simulink model "Distribution_vAggregate"  (Simulink 7.9)
settings: Solver=VariableStepDiscrete  StartTime=0.0  StopTime=1000  RelTol=1e-3
libraries: simeventslib x23
(part 1 of 4)
settings Model: Creator=tsprock3  LastModifiedBy=tsprock3
settings DebuggingCC: SimStateOlderReleaseMsg=warning

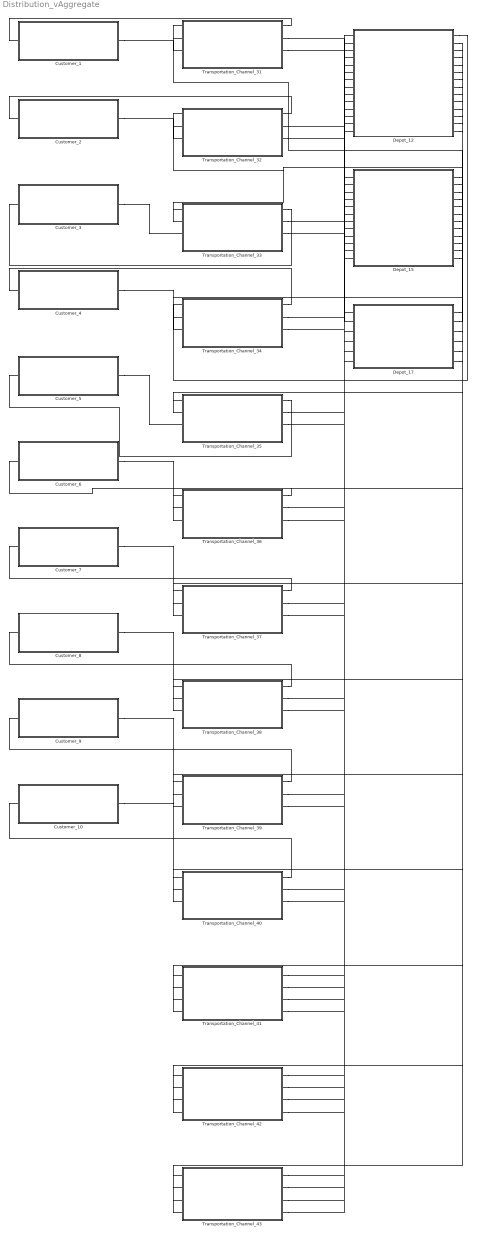
== system Distribution_vAggregate ==
  Customer_1 : Subsystem
  Customer_10 : Subsystem
  Customer_2 : Subsystem
  Customer_3 : Subsystem
  Customer_4 : Subsystem
  Customer_5 : Subsystem
  Customer_6 : Subsystem
  Customer_7 : Subsystem
  Customer_8 : Subsystem
  Customer_9 : Subsystem
  Depot_12 : Subsystem
  Depot_15 : Subsystem
  Depot_17 : Subsystem
  Transportation_Channel_31 : Subsystem
  Transportation_Channel_32 : Subsystem
  Transportation_Channel_33 : Subsystem
  Transportation_Channel_34 : Subsystem
  Transportation_Channel_35 : Subsystem
  Transportation_Channel_36 : Subsystem
  Transportation_Channel_37 : Subsystem
  Transportation_Channel_38 : Subsystem
  Transportation_Channel_39 : Subsystem
  Transportation_Channel_40 : Subsystem
  Transportation_Channel_41 : Subsystem
  Transportation_Channel_42 : Subsystem
  Transportation_Channel_43 : Subsystem
  connections:
  Depot_17/RConn1 -- Transportation_Channel_31/LConn1
  Transportation_Channel_31/RConn1 -- Customer_1/LConn1
  Depot_17/RConn2 -- Transportation_Channel_31/LConn2
  Transportation_Channel_31/RConn2 -- Depot_17/LConn1
  Customer_1/RConn1 -- Transportation_Channel_31/LConn3
  Transportation_Channel_31/RConn3 -- Depot_17/LConn2
  Depot_15/RConn1 -- Transportation_Channel_32/LConn1
  Transportation_Channel_32/RConn1 -- Customer_2/LConn1
  Depot_15/RConn2 -- Transportation_Channel_32/LConn2
  Transportation_Channel_32/RConn2 -- Depot_15/LConn1
  Customer_2/RConn1 -- Transportation_Channel_32/LConn3
  Transportation_Channel_32/RConn3 -- Depot_15/LConn2
  Depot_15/RConn3 -- Transportation_Channel_33/LConn1
  Transportation_Channel_33/RConn1 -- Customer_3/LConn1
  Depot_15/RConn4 -- Transportation_Channel_33/LConn2
  Transportation_Channel_33/RConn2 -- Depot_15/LConn3
  Customer_3/RConn1 -- Transportation_Channel_33/LConn3
  Transportation_Channel_33/RConn3 -- Depot_15/LConn4
  Depot_12/RConn1 -- Transportation_Channel_34/LConn1
  Transportation_Channel_34/RConn1 -- Customer_4/LConn1
  Depot_12/RConn2 -- Transportation_Channel_34/LConn2
  Transportation_Channel_34/RConn2 -- Depot_12/LConn1
  Customer_4/RConn1 -- Transportation_Channel_34/LConn3
  Transportation_Channel_34/RConn3 -- Depot_12/LConn2
  Depot_12/RConn3 -- Transportation_Channel_35/LConn1
  Transportation_Channel_35/RConn1 -- Customer_5/LConn1
  Depot_12/RConn4 -- Transportation_Channel_35/LConn2
  Transportation_Channel_35/RConn2 -- Depot_12/LConn3
  Customer_5/RConn1 -- Transportation_Channel_35/LConn3
  Transportation_Channel_35/RConn3 -- Depot_12/LConn4
  Depot_12/RConn5 -- Transportation_Channel_36/LConn1
  Transportation_Channel_36/RConn1 -- Customer_6/LConn1
  Depot_12/RConn6 -- Transportation_Channel_36/LConn2
  Transportation_Channel_36/RConn2 -- Depot_12/LConn5
  Customer_6/RConn1 -- Transportation_Channel_36/LConn3
  Transportation_Channel_36/RConn3 -- Depot_12/LConn6
  Depot_12/RConn7 -- Transportation_Channel_37/LConn1
  Transportation_Channel_37/RConn1 -- Customer_7/LConn1
  Depot_12/RConn8 -- Transportation_Channel_37/LConn2
  Transportation_Channel_37/RConn2 -- Depot_12/LConn7
  Customer_7/RConn1 -- Transportation_Channel_37/LConn3
  Transportation_Channel_37/RConn3 -- Depot_12/LConn8
  Depot_15/RConn5 -- Transportation_Channel_38/LConn1
  Transportation_Channel_38/RConn1 -- Customer_8/LConn1
  Depot_15/RConn6 -- Transportation_Channel_38/LConn2
  Transportation_Channel_38/RConn2 -- Depot_15/LConn5
  Customer_8/RConn1 -- Transportation_Channel_38/LConn3
  Transportation_Channel_38/RConn3 -- Depot_15/LConn6
  Depot_15/RConn7 -- Transportation_Channel_39/LConn1
  Transportation_Channel_39/RConn1 -- Customer_9/LConn1
  Depot_15/RConn8 -- Transportation_Channel_39/LConn2
  Transportation_Channel_39/RConn2 -- Depot_15/LConn7
  Customer_9/RConn1 -- Transportation_Channel_39/LConn3
  Transportation_Channel_39/RConn3 -- Depot_15/LConn8
  Depot_12/RConn9 -- Transportation_Channel_40/LConn1
  Transportation_Channel_40/RConn1 -- Customer_10/LConn1
  Depot_12/RConn10 -- Transportation_Channel_40/LConn2
  Transportation_Channel_40/RConn2 -- Depot_12/LConn9
  Customer_10/RConn1 -- Transportation_Channel_40/LConn3
  Transportation_Channel_40/RConn3 -- Depot_12/LConn10
  Depot_15/RConn9 -- Transportation_Channel_41/LConn1
  Transportation_Channel_41/RConn1 -- Depot_12/LConn11
  Depot_15/RConn10 -- Transportation_Channel_41/LConn2
  Transportation_Channel_41/RConn2 -- Depot_15/LConn9
  Depot_12/RConn11 -- Transportation_Channel_41/LConn3
  Transportation_Channel_41/RConn3 -- Depot_15/LConn10
  Depot_12/RConn12 -- Transportation_Channel_41/LConn4
  Transportation_Channel_41/RConn4 -- Depot_12/LConn12
  Depot_17/RConn3 -- Transportation_Channel_42/LConn1
  Transportation_Channel_42/RConn1 -- Depot_12/LConn13
  Depot_17/RConn4 -- Transportation_Channel_42/LConn2
  Transportation_Channel_42/RConn2 -- Depot_17/LConn3
  Depot_12/RConn13 -- Transportation_Channel_42/LConn3
  Transportation_Channel_42/RConn3 -- Depot_17/LConn4
  Depot_12/RConn14 -- Transportation_Channel_42/LConn4
  Transportation_Channel_42/RConn4 -- Depot_12/LConn14
  Depot_17/RConn5 -- Transportation_Channel_43/LConn1
  Transportation_Channel_43/RConn1 -- Depot_15/LConn11
  Depot_17/RConn6 -- Transportation_Channel_43/LConn2
  Transportation_Channel_43/RConn2 -- Depot_17/LConn5
  Depot_15/RConn11 -- Transportation_Channel_43/LConn3
  Transportation_Channel_43/RConn3 -- Depot_17/LConn6
  Depot_15/RConn12 -- Transportation_Channel_43/LConn4
  Transportation_Channel_43/RConn4 -- Depot_15/LConn12

== system Distribution_vAggregate/Customer_1 ==
  Commodity_1 : Subsystem  mask{Mean=2000/340, AttributeValue=[1  17  15   2   0   0]|1|2|1}
      mask prompts: Mean "Frequency"; AttributeValue "Attributes"
  Commodity_2 : Subsystem  mask{Mean=2000/473, AttributeValue=[1  17  15   3   0   0]|1|3|1}
      mask prompts: Mean "Frequency"; AttributeValue "Attributes"
  Commodity_3 : Subsystem  mask{Mean=2000/355, AttributeValue=[1  17  12   4   0   0]|1|4|1}
      mask prompts: Mean "Frequency"; AttributeValue "Attributes"
  Commodity_4 : Subsystem  mask{Mean=2000/60, AttributeValue=[1  17  12   5   0   0]|1|5|1}
      mask prompts: Mean "Frequency"; AttributeValue "Attributes"
  Commodity_5 : Subsystem  mask{Mean=2000/226, AttributeValue=[1  17  12   6   0   0]|1|6|1}
      mask prompts: Mean "Frequency"; AttributeValue "Attributes"
  Commodity_6 : Subsystem  mask{Mean=2000/331, AttributeValue=[1  17  12   7   0   0]|1|7|1}
      mask prompts: Mean "Frequency"; AttributeValue "Attributes"
  Commodity_7 : Subsystem  mask{Mean=2000/176, AttributeValue=[1  17  15   8   0   0]|1|8|1}
      mask prompts: Mean "Frequency"; AttributeValue "Attributes"
  Commodity_8 : Subsystem  mask{Mean=2000/209, AttributeValue=[1  17  15   9   0   0]|1|9|1}
      mask prompts: Mean "Frequency"; AttributeValue "Attributes"
  Commodity_9 : Subsystem  mask{Mean=2000/417, AttributeValue=[1  17  12  10   0   0]|1|10|1}
      mask prompts: Mean "Frequency"; AttributeValue "Attributes"
  Entity Sink : EntitySink
  Get Attribute : GetAttribute  AttributeName=Origin|Destination|Start  AttributeMissing=Error|Error|Error  AttributeDefaultValue=1|1|1  AttributeTreatAsVector=1|1|1  AttributeSendTiming=After entity departure|After entity departure|After entity departure  EvaluatedDefaultAttributeValue={[];[];[]}
      settings: OutputPortMap=o1,o2,o3
  Get Attribute1 : GetAttribute  AttributeName=Route  EvaluatedDefaultAttributeValue={[]}
      settings: OutputPortMap=o1
  IN_Commodity : PathCombiner  NumberInputPorts=9
  IN_Shipment : PathCombiner  NumberInputPorts=1
  Lookup : Constant  Value=[17]
  MATLAB Function : MATLAB Function  TreatAsAtomicUnit=on
  Mux : Mux  Inputs=3
  Node_ID : Constant
  OUT_Shipment : OutputSwitch  NumberOutputPorts=1  SwitchingCriterion=From signal port p  AttributeName=Customer
  Shipment_Metrics : simeventslib/SimEvents Sinks/Discrete Event Signal to Workspace  VariableName=Customer_1  SaveFormat=Structure With Time  isMonitorOnly=off  isRecordIC=off
  Single Server : SingleServer  ServiceTime=0
  Timed to Evnt Signal : TimedToEventSignal
  Timed to Evnt Signal1 : TimedToEventSignal
  IN_Shipment_1 : PMIOPort  Port=1  Side=Left
  OUT_Shipment_1 : PMIOPort  Port=2  Side=Right
  wires:
  Timed to Evnt Signal1/1 -> MATLAB Function/3(lookup)
  Lookup/1 -> Timed to Evnt Signal1/1
  Timed to Evnt Signal/1 -> MATLAB Function/2(current)
  Get Attribute1/1 -> MATLAB Function/1(route)
  MATLAB Function/1(next) -> OUT_Shipment/1
  Node_ID/1 -> Timed to Evnt Signal/1
  Mux/1 -> Shipment_Metrics/1
  Get Attribute/3 -> Mux/3
  Get Attribute/2 -> Mux/2
  Get Attribute/1 -> Mux/1
  connections:
  Single Server/RConn1 -- OUT_Shipment/LConn1
  Get Attribute1/RConn1 -- Single Server/LConn1
  IN_Commodity/RConn1 -- Get Attribute1/LConn1
  Get Attribute/LConn1 -- IN_Shipment/RConn1
  Entity Sink/LConn1 -- Get Attribute/RConn1
  IN_Shipment/LConn1 -- IN_Shipment_1/RConn1
  OUT_Shipment/RConn1 -- OUT_Shipment_1/RConn1
  Commodity_1/RConn1 -- IN_Commodity/LConn1
  Commodity_2/RConn1 -- IN_Commodity/LConn2
  Commodity_3/RConn1 -- IN_Commodity/LConn3
  Commodity_4/RConn1 -- IN_Commodity/LConn4
  Commodity_5/RConn1 -- IN_Commodity/LConn5
  Commodity_6/RConn1 -- IN_Commodity/LConn6
  Commodity_7/RConn1 -- IN_Commodity/LConn7
  Commodity_8/RConn1 -- IN_Commodity/LConn8
  Commodity_9/RConn1 -- IN_Commodity/LConn9

== system Distribution_vAggregate/Customer_10 ==
  Commodity_82 : Subsystem  mask{Mean=2000/308, AttributeValue=[10  12  17   1   0   0]|10|1|1}
      mask prompts: Mean "Frequency"; AttributeValue "Attributes"
  Commodity_83 : Subsystem  mask{Mean=2000/25, AttributeValue=[10  12  15   2   0   0]|10|2|1}
      mask prompts: Mean "Frequency"; AttributeValue "Attributes"
  Commodity_84 : Subsystem  mask{Mean=2000/97, AttributeValue=[10  12  15   3   0   0]|10|3|1}
      mask prompts: Mean "Frequency"; AttributeValue "Attributes"
  Commodity_85 : Subsystem  mask{Mean=2000/103, AttributeValue=[10  12   4   0   0   0]|10|4|1}
      mask prompts: Mean "Frequency"; AttributeValue "Attributes"
  Commodity_86 : Subsystem  mask{Mean=2000/95, AttributeValue=[10  12   5   0   0   0]|10|5|1}
      mask prompts: Mean "Frequency"; AttributeValue "Attributes"
  Commodity_87 : Subsystem  mask{Mean=2000/318, AttributeValue=[10  12   6   0   0   0]|10|6|1}
      mask prompts: Mean "Frequency"; AttributeValue "Attributes"
  Commodity_88 : Subsystem  mask{Mean=2000/270, AttributeValue=[10  12   7   0   0   0]|10|7|1}
      mask prompts: Mean "Frequency"; AttributeValue "Attributes"
  Commodity_89 : Subsystem  mask{Mean=2000/250, AttributeValue=[10  12  15   8   0   0]|10|8|1}
      mask prompts: Mean "Frequency"; AttributeValue "Attributes"
  Commodity_90 : Subsystem  mask{Mean=2000/223, AttributeValue=[10  12  15   9   0   0]|10|9|1}
      mask prompts: Mean "Frequency"; AttributeValue "Attributes"
  Entity Sink : EntitySink
  Get Attribute : GetAttribute  AttributeName=Origin|Destination|Start  AttributeMissing=Error|Error|Error  AttributeDefaultValue=1|1|1  AttributeTreatAsVector=1|1|1  AttributeSendTiming=After entity departure|After entity departure|After entity departure  EvaluatedDefaultAttributeValue={[];[];[]}
      settings: OutputPortMap=o1,o2,o3
  Get Attribute1 : GetAttribute  AttributeName=Route  EvaluatedDefaultAttributeValue={[]}
      settings: OutputPortMap=o1
  IN_Commodity : PathCombiner  NumberInputPorts=9
  IN_Shipment : PathCombiner  NumberInputPorts=1
  Lookup : Constant  Value=[12]
  MATLAB Function : MATLAB Function  TreatAsAtomicUnit=on
  Mux : Mux  Inputs=3
  Node_ID : Constant  Value=10
  OUT_Shipment : OutputSwitch  NumberOutputPorts=1  SwitchingCriterion=From signal port p  AttributeName=Customer
  Shipment_Metrics : simeventslib/SimEvents Sinks/Discrete Event Signal to Workspace  VariableName=Customer_10  SaveFormat=Structure With Time  isMonitorOnly=off  isRecordIC=off
  Single Server : SingleServer  ServiceTime=0
  Timed to Evnt Signal : TimedToEventSignal
  Timed to Evnt Signal1 : TimedToEventSignal
  IN_Shipment_1 : PMIOPort  Port=1  Side=Left
  OUT_Shipment_1 : PMIOPort  Port=2  Side=Right
  wires:
  Timed to Evnt Signal1/1 -> MATLAB Function/3(lookup)
  Lookup/1 -> Timed to Evnt Signal1/1
  Timed to Evnt Signal/1 -> MATLAB Function/2(current)
  Get Attribute1/1 -> MATLAB Function/1(route)
  MATLAB Function/1(next) -> OUT_Shipment/1
  Node_ID/1 -> Timed to Evnt Signal/1
  Mux/1 -> Shipment_Metrics/1
  Get Attribute/3 -> Mux/3
  Get Attribute/2 -> Mux/2
  Get Attribute/1 -> Mux/1
  connections:
  Single Server/RConn1 -- OUT_Shipment/LConn1
  Get Attribute1/RConn1 -- Single Server/LConn1
  IN_Commodity/RConn1 -- Get Attribute1/LConn1
  Get Attribute/LConn1 -- IN_Shipment/RConn1
  Entity Sink/LConn1 -- Get Attribute/RConn1
  IN_Shipment/LConn1 -- IN_Shipment_1/RConn1
  OUT_Shipment/RConn1 -- OUT_Shipment_1/RConn1
  Commodity_82/RConn1 -- IN_Commodity/LConn1
  Commodity_83/RConn1 -- IN_Commodity/LConn2
  Commodity_84/RConn1 -- IN_Commodity/LConn3
  Commodity_85/RConn1 -- IN_Commodity/LConn4
  Commodity_86/RConn1 -- IN_Commodity/LConn5
  Commodity_87/RConn1 -- IN_Commodity/LConn6
  Commodity_88/RConn1 -- IN_Commodity/LConn7
  Commodity_89/RConn1 -- IN_Commodity/LConn8
  Commodity_90/RConn1 -- IN_Commodity/LConn9

== system Distribution_vAggregate/Customer_2 ==
  Commodity_10 : Subsystem  mask{Mean=2000/307, AttributeValue=[2  15  17   1   0   0]|2|1|1}
      mask prompts: Mean "Frequency"; AttributeValue "Attributes"
  Commodity_11 : Subsystem  mask{Mean=2000/271, AttributeValue=[2  15   3   0   0   0]|2|3|1}
      mask prompts: Mean "Frequency"; AttributeValue "Attributes"
  Commodity_12 : Subsystem  mask{Mean=2000/133, AttributeValue=[2  15  12   4   0   0]|2|4|1}
      mask prompts: Mean "Frequency"; AttributeValue "Attributes"
  Commodity_13 : Subsystem  mask{Mean=2000/60, AttributeValue=[2  15  12   5   0   0]|2|5|1}
      mask prompts: Mean "Frequency"; AttributeValue "Attributes"
  Commodity_14 : Subsystem  mask{Mean=2000/323, AttributeValue=[2  15  12   6   0   0]|2|6|1}
      mask prompts: Mean "Frequency"; AttributeValue "Attributes"
  Commodity_15 : Subsystem  mask{Mean=2000/320, AttributeValue=[2  15  12   7   0   0]|2|7|1}
      mask prompts: Mean "Frequency"; AttributeValue "Attributes"
  Commodity_16 : Subsystem  mask{Mean=2000/324, AttributeValue=[2  15   8   0   0   0]|2|8|1}
      mask prompts: Mean "Frequency"; AttributeValue "Attributes"
  Commodity_17 : Subsystem  mask{Mean=2000/361, AttributeValue=[2  15   9   0   0   0]|2|9|1}
      mask prompts: Mean "Frequency"; AttributeValue "Attributes"
  Commodity_18 : Subsystem  mask{Mean=2000/497, AttributeValue=[2  15  12  10   0   0]|2|10|1}
      mask prompts: Mean "Frequency"; AttributeValue "Attributes"
  Entity Sink : EntitySink
  Get Attribute : GetAttribute  AttributeName=Origin|Destination|Start  AttributeMissing=Error|Error|Error  AttributeDefaultValue=1|1|1  AttributeTreatAsVector=1|1|1  AttributeSendTiming=After entity departure|After entity departure|After entity departure  EvaluatedDefaultAttributeValue={[];[];[]}
      settings: OutputPortMap=o1,o2,o3
  Get Attribute1 : GetAttribute  AttributeName=Route  EvaluatedDefaultAttributeValue={[]}
      settings: OutputPortMap=o1
  IN_Commodity : PathCombiner  NumberInputPorts=9
  IN_Shipment : PathCombiner  NumberInputPorts=1
  Lookup : Constant  Value=[15]
  MATLAB Function : MATLAB Function  TreatAsAtomicUnit=on
  Mux : Mux  Inputs=3
  Node_ID : Constant  Value=2
  OUT_Shipment : OutputSwitch  NumberOutputPorts=1  SwitchingCriterion=From signal port p  AttributeName=Customer
  Shipment_Metrics : simeventslib/SimEvents Sinks/Discrete Event Signal to Workspace  VariableName=Customer_2  SaveFormat=Structure With Time  isMonitorOnly=off  isRecordIC=off
  Single Server : SingleServer  ServiceTime=0
  Timed to Evnt Signal : TimedToEventSignal
  Timed to Evnt Signal1 : TimedToEventSignal
  IN_Shipment_1 : PMIOPort  Port=1  Side=Left
  OUT_Shipment_1 : PMIOPort  Port=2  Side=Right
  wires:
  Timed to Evnt Signal1/1 -> MATLAB Function/3(lookup)
  Lookup/1 -> Timed to Evnt Signal1/1
  Timed to Evnt Signal/1 -> MATLAB Function/2(current)
  Get Attribute1/1 -> MATLAB Function/1(route)
  MATLAB Function/1(next) -> OUT_Shipment/1
  Node_ID/1 -> Timed to Evnt Signal/1
  Mux/1 -> Shipment_Metrics/1
  Get Attribute/3 -> Mux/3
  Get Attribute/2 -> Mux/2
  Get Attribute/1 -> Mux/1
  connections:
  Single Server/RConn1 -- OUT_Shipment/LConn1
  Get Attribute1/RConn1 -- Single Server/LConn1
  IN_Commodity/RConn1 -- Get Attribute1/LConn1
  Get Attribute/LConn1 -- IN_Shipment/RConn1
  Entity Sink/LConn1 -- Get Attribute/RConn1
  IN_Shipment/LConn1 -- IN_Shipment_1/RConn1
  OUT_Shipment/RConn1 -- OUT_Shipment_1/RConn1
  Commodity_10/RConn1 -- IN_Commodity/LConn1
  Commodity_11/RConn1 -- IN_Commodity/LConn2
  Commodity_12/RConn1 -- IN_Commodity/LConn3
  Commodity_13/RConn1 -- IN_Commodity/LConn4
  Commodity_14/RConn1 -- IN_Commodity/LConn5
  Commodity_15/RConn1 -- IN_Commodity/LConn6
  Commodity_16/RConn1 -- IN_Commodity/LConn7
  Commodity_17/RConn1 -- IN_Commodity/LConn8
  Commodity_18/RConn1 -- IN_Commodity/LConn9

== system Distribution_vAggregate/Customer_3 ==
  Commodity_19 : Subsystem  mask{Mean=2000/53, AttributeValue=[3  15  17   1   0   0]|3|1|1}
      mask prompts: Mean "Frequency"; AttributeValue "Attributes"
  Commodity_20 : Subsystem  mask{Mean=2000/32, AttributeValue=[3  15   2   0   0   0]|3|2|1}
      mask prompts: Mean "Frequency"; AttributeValue "Attributes"
  Commodity_21 : Subsystem  mask{Mean=2000/225, AttributeValue=[3  15  12   4   0   0]|3|4|1}
      mask prompts: Mean "Frequency"; AttributeValue "Attributes"
  Commodity_22 : Subsystem  mask{Mean=2000/382, AttributeValue=[3  15  12   5   0   0]|3|5|1}
      mask prompts: Mean "Frequency"; AttributeValue "Attributes"
  Commodity_23 : Subsystem  mask{Mean=2000/386, AttributeValue=[3  15  12   6   0   0]|3|6|1}
      mask prompts: Mean "Frequency"; AttributeValue "Attributes"
  Commodity_24 : Subsystem  mask{Mean=2000/487, AttributeValue=[3  15  12   7   0   0]|3|7|1}
      mask prompts: Mean "Frequency"; AttributeValue "Attributes"
  Commodity_25 : Subsystem  mask{Mean=2000/70, AttributeValue=[3  15   8   0   0   0]|3|8|1}
      mask prompts: Mean "Frequency"; AttributeValue "Attributes"
  Commodity_26 : Subsystem  mask{Mean=2000/47, AttributeValue=[3  15   9   0   0   0]|3|9|1}
      mask prompts: Mean "Frequency"; AttributeValue "Attributes"
  Commodity_27 : Subsystem  mask{Mean=2000/266, AttributeValue=[3  15  12  10   0   0]|3|10|1}
      mask prompts: Mean "Frequency"; AttributeValue "Attributes"
  Entity Sink : EntitySink
  Get Attribute : GetAttribute  AttributeName=Origin|Destination|Start  AttributeMissing=Error|Error|Error  AttributeDefaultValue=1|1|1  AttributeTreatAsVector=1|1|1  AttributeSendTiming=After entity departure|After entity departure|After entity departure  EvaluatedDefaultAttributeValue={[];[];[]}
      settings: OutputPortMap=o1,o2,o3
  Get Attribute1 : GetAttribute  AttributeName=Route  EvaluatedDefaultAttributeValue={[]}
      settings: OutputPortMap=o1
  IN_Commodity : PathCombiner  NumberInputPorts=9
  IN_Shipment : PathCombiner  NumberInputPorts=1
  Lookup : Constant  Value=[15]
  MATLAB Function : MATLAB Function  TreatAsAtomicUnit=on
  Mux : Mux  Inputs=3
  Node_ID : Constant  Value=3
  OUT_Shipment : OutputSwitch  NumberOutputPorts=1  SwitchingCriterion=From signal port p  AttributeName=Customer
  Shipment_Metrics : simeventslib/SimEvents Sinks/Discrete Event Signal to Workspace  VariableName=Customer_3  SaveFormat=Structure With Time  isMonitorOnly=off  isRecordIC=off
  Single Server : SingleServer  ServiceTime=0
  Timed to Evnt Signal : TimedToEventSignal
  Timed to Evnt Signal1 : TimedToEventSignal
  IN_Shipment_1 : PMIOPort  Port=1  Side=Left
  OUT_Shipment_1 : PMIOPort  Port=2  Side=Right
  wires:
  Timed to Evnt Signal1/1 -> MATLAB Function/3(lookup)
  Lookup/1 -> Timed to Evnt Signal1/1
  Timed to Evnt Signal/1 -> MATLAB Function/2(current)
  Get Attribute1/1 -> MATLAB Function/1(route)
  MATLAB Function/1(next) -> OUT_Shipment/1
  Node_ID/1 -> Timed to Evnt Signal/1
  Mux/1 -> Shipment_Metrics/1
  Get Attribute/3 -> Mux/3
  Get Attribute/2 -> Mux/2
  Get Attribute/1 -> Mux/1
  connections:
  Single Server/RConn1 -- OUT_Shipment/LConn1
  Get Attribute1/RConn1 -- Single Server/LConn1
  IN_Commodity/RConn1 -- Get Attribute1/LConn1
  Get Attribute/LConn1 -- IN_Shipment/RConn1
  Entity Sink/LConn1 -- Get Attribute/RConn1
  IN_Shipment/LConn1 -- IN_Shipment_1/RConn1
  OUT_Shipment/RConn1 -- OUT_Shipment_1/RConn1
  Commodity_19/RConn1 -- IN_Commodity/LConn1
  Commodity_20/RConn1 -- IN_Commodity/LConn2
  Commodity_21/RConn1 -- IN_Commodity/LConn3
  Commodity_22/RConn1 -- IN_Commodity/LConn4
  Commodity_23/RConn1 -- IN_Commodity/LConn5
  Commodity_24/RConn1 -- IN_Commodity/LConn6
  Commodity_25/RConn1 -- IN_Commodity/LConn7
  Commodity_26/RConn1 -- IN_Commodity/LConn8
  Commodity_27/RConn1 -- IN_Commodity/LConn9

== system Distribution_vAggregate/Customer_4 ==
  Commodity_28 : Subsystem  mask{Mean=2000/243, AttributeValue=[4  12  17   1   0   0]|4|1|1}
      mask prompts: Mean "Frequency"; AttributeValue "Attributes"
  Commodity_29 : Subsystem  mask{Mean=2000/336, AttributeValue=[4  12  15   2   0   0]|4|2|1}
      mask prompts: Mean "Frequency"; AttributeValue "Attributes"
  Commodity_30 : Subsystem  mask{Mean=2000/261, AttributeValue=[4  12  15   3   0   0]|4|3|1}
      mask prompts: Mean "Frequency"; AttributeValue "Attributes"
  Commodity_31 : Subsystem  mask{Mean=2000/75, AttributeValue=[4  12   5   0   0   0]|4|5|1}
      mask prompts: Mean "Frequency"; AttributeValue "Attributes"
  Commodity_32 : Subsystem  mask{Mean=2000/132, AttributeValue=[4  12   6   0   0   0]|4|6|1}
      mask prompts: Mean "Frequency"; AttributeValue "Attributes"
  Commodity_33 : Subsystem  mask{Mean=2000/378, AttributeValue=[4  12   7   0   0   0]|4|7|1}
      mask prompts: Mean "Frequency"; AttributeValue "Attributes"
  Commodity_34 : Subsystem  mask{Mean=2000/222, AttributeValue=[4  12  15   8   0   0]|4|8|1}
      mask prompts: Mean "Frequency"; AttributeValue "Attributes"
  Commodity_35 : Subsystem  mask{Mean=2000/180, AttributeValue=[4  12  15   9   0   0]|4|9|1}
      mask prompts: Mean "Frequency"; AttributeValue "Attributes"
  Commodity_36 : Subsystem  mask{Mean=2000/198, AttributeValue=[4  12  10   0   0   0]|4|10|1}
      mask prompts: Mean "Frequency"; AttributeValue "Attributes"
  Entity Sink : EntitySink
  Get Attribute : GetAttribute  AttributeName=Origin|Destination|Start  AttributeMissing=Error|Error|Error  AttributeDefaultValue=1|1|1  AttributeTreatAsVector=1|1|1  AttributeSendTiming=After entity departure|After entity departure|After entity departure  EvaluatedDefaultAttributeValue={[];[];[]}
      settings: OutputPortMap=o1,o2,o3
  Get Attribute1 : GetAttribute  AttributeName=Route  EvaluatedDefaultAttributeValue={[]}
      settings: OutputPortMap=o1
  IN_Commodity : PathCombiner  NumberInputPorts=9
  IN_Shipment : PathCombiner  NumberInputPorts=1
  Lookup : Constant  Value=[12]
  MATLAB Function : MATLAB Function  TreatAsAtomicUnit=on
  Mux : Mux  Inputs=3
  Node_ID : Constant  Value=4
  OUT_Shipment : OutputSwitch  NumberOutputPorts=1  SwitchingCriterion=From signal port p  AttributeName=Customer
  Shipment_Metrics : simeventslib/SimEvents Sinks/Discrete Event Signal to Workspace  VariableName=Customer_4  SaveFormat=Structure With Time  isMonitorOnly=off  isRecordIC=off
  Single Server : SingleServer  ServiceTime=0
  Timed to Evnt Signal : TimedToEventSignal
  Timed to Evnt Signal1 : TimedToEventSignal
  IN_Shipment_1 : PMIOPort  Port=1  Side=Left
  OUT_Shipment_1 : PMIOPort  Port=2  Side=Right
  wires:
  Timed to Evnt Signal1/1 -> MATLAB Function/3(lookup)
  Lookup/1 -> Timed to Evnt Signal1/1
  Timed to Evnt Signal/1 -> MATLAB Function/2(current)
  Get Attribute1/1 -> MATLAB Function/1(route)
  MATLAB Function/1(next) -> OUT_Shipment/1
  Node_ID/1 -> Timed to Evnt Signal/1
  Mux/1 -> Shipment_Metrics/1
  Get Attribute/3 -> Mux/3
  Get Attribute/2 -> Mux/2
  Get Attribute/1 -> Mux/1
  connections:
  Single Server/RConn1 -- OUT_Shipment/LConn1
  Get Attribute1/RConn1 -- Single Server/LConn1
  IN_Commodity/RConn1 -- Get Attribute1/LConn1
  Get Attribute/LConn1 -- IN_Shipment/RConn1
  Entity Sink/LConn1 -- Get Attribute/RConn1
  IN_Shipment/LConn1 -- IN_Shipment_1/RConn1
  OUT_Shipment/RConn1 -- OUT_Shipment_1/RConn1
  Commodity_28/RConn1 -- IN_Commodity/LConn1
  Commodity_29/RConn1 -- IN_Commodity/LConn2
  Commodity_30/RConn1 -- IN_Commodity/LConn3
  Commodity_31/RConn1 -- IN_Commodity/LConn4
  Commodity_32/RConn1 -- IN_Commodity/LConn5
  Commodity_33/RConn1 -- IN_Commodity/LConn6
  Commodity_34/RConn1 -- IN_Commodity/LConn7
  Commodity_35/RConn1 -- IN_Commodity/LConn8
  Commodity_36/RConn1 -- IN_Commodity/LConn9

== system Distribution_vAggregate/Customer_5 ==
  Commodity_37 : Subsystem  mask{Mean=2000/353, AttributeValue=[5  12  17   1   0   0]|5|1|1}
      mask prompts: Mean "Frequency"; AttributeValue "Attributes"
  Commodity_38 : Subsystem  mask{Mean=2000/10, AttributeValue=[5  12  15   2   0   0]|5|2|1}
      mask prompts: Mean "Frequency"; AttributeValue "Attributes"
  Commodity_39 : Subsystem  mask{Mean=2000/213, AttributeValue=[5  12  15   3   0   0]|5|3|1}
      mask prompts: Mean "Frequency"; AttributeValue "Attributes"
  Commodity_40 : Subsystem  mask{Mean=2000/99, AttributeValue=[5  12   4   0   0   0]|5|4|1}
      mask prompts: Mean "Frequency"; AttributeValue "Attributes"
  Commodity_41 : Subsystem  mask{Mean=2000/215, AttributeValue=[5  12   6   0   0   0]|5|6|1}
      mask prompts: Mean "Frequency"; AttributeValue "Attributes"
  Commodity_42 : Subsystem  mask{Mean=2000/196, AttributeValue=[5  12   7   0   0   0]|5|7|1}
      mask prompts: Mean "Frequency"; AttributeValue "Attributes"
  Commodity_43 : Subsystem  mask{Mean=2000/199, AttributeValue=[5  12  15   8   0   0]|5|8|1}
      mask prompts: Mean "Frequency"; AttributeValue "Attributes"
  Commodity_44 : Subsystem  mask{Mean=2000/378, AttributeValue=[5  12  15   9   0   0]|5|9|1}
      mask prompts: Mean "Frequency"; AttributeValue "Attributes"
  Commodity_45 : Subsystem  mask{Mean=2000/109, AttributeValue=[5  12  10   0   0   0]|5|10|1}
      mask prompts: Mean "Frequency"; AttributeValue "Attributes"
  Entity Sink : EntitySink
  Get Attribute : GetAttribute  AttributeName=Origin|Destination|Start  AttributeMissing=Error|Error|Error  AttributeDefaultValue=1|1|1  AttributeTreatAsVector=1|1|1  AttributeSendTiming=After entity departure|After entity departure|After entity departure  EvaluatedDefaultAttributeValue={[];[];[]}
      settings: OutputPortMap=o1,o2,o3
  Get Attribute1 : GetAttribute  AttributeName=Route  EvaluatedDefaultAttributeValue={[]}
      settings: OutputPortMap=o1
  IN_Commodity : PathCombiner  NumberInputPorts=9
  IN_Shipment : PathCombiner  NumberInputPorts=1
  Lookup : Constant  Value=[12]
  MATLAB Function : MATLAB Function  TreatAsAtomicUnit=on
  Mux : Mux  Inputs=3
  Node_ID : Constant  Value=5
  OUT_Shipment : OutputSwitch  NumberOutputPorts=1  SwitchingCriterion=From signal port p  AttributeName=Customer
  Shipment_Metrics : simeventslib/SimEvents Sinks/Discrete Event Signal to Workspace  VariableName=Customer_5  SaveFormat=Structure With Time  isMonitorOnly=off  isRecordIC=off
  Single Server : SingleServer  ServiceTime=0
  Timed to Evnt Signal : TimedToEventSignal
  Timed to Evnt Signal1 : TimedToEventSignal
  IN_Shipment_1 : PMIOPort  Port=1  Side=Left
  OUT_Shipment_1 : PMIOPort  Port=2  Side=Right
  wires:
  Timed to Evnt Signal1/1 -> MATLAB Function/3(lookup)
  Lookup/1 -> Timed to Evnt Signal1/1
  Timed to Evnt Signal/1 -> MATLAB Function/2(current)
  Get Attribute1/1 -> MATLAB Function/1(route)
  MATLAB Function/1(next) -> OUT_Shipment/1
  Node_ID/1 -> Timed to Evnt Signal/1
  Mux/1 -> Shipment_Metrics/1
  Get Attribute/3 -> Mux/3
  Get Attribute/2 -> Mux/2
  Get Attribute/1 -> Mux/1
  connections:
  Single Server/RConn1 -- OUT_Shipment/LConn1
  Get Attribute1/RConn1 -- Single Server/LConn1
  IN_Commodity/RConn1 -- Get Attribute1/LConn1
  Get Attribute/LConn1 -- IN_Shipment/RConn1
  Entity Sink/LConn1 -- Get Attribute/RConn1
  IN_Shipment/LConn1 -- IN_Shipment_1/RConn1
  OUT_Shipment/RConn1 -- OUT_Shipment_1/RConn1
  Commodity_37/RConn1 -- IN_Commodity/LConn1
  Commodity_38/RConn1 -- IN_Commodity/LConn2
  Commodity_39/RConn1 -- IN_Commodity/LConn3
  Commodity_40/RConn1 -- IN_Commodity/LConn4
  Commodity_41/RConn1 -- IN_Commodity/LConn5
  Commodity_42/RConn1 -- IN_Commodity/LConn6
  Commodity_43/RConn1 -- IN_Commodity/LConn7
  Commodity_44/RConn1 -- IN_Commodity/LConn8
  Commodity_45/RConn1 -- IN_Commodity/LConn9

== system Distribution_vAggregate/Customer_6 ==
  Commodity_46 : Subsystem  mask{Mean=2000/475, AttributeValue=[6  12  17   1   0   0]|6|1|1}
      mask prompts: Mean "Frequency"; AttributeValue "Attributes"
  Commodity_47 : Subsystem  mask{Mean=2000/336, AttributeValue=[6  12  15   2   0   0]|6|2|1}
      mask prompts: Mean "Frequency"; AttributeValue "Attributes"
  Commodity_48 : Subsystem  mask{Mean=2000/417, AttributeValue=[6  12  15   3   0   0]|6|3|1}
      mask prompts: Mean "Frequency"; AttributeValue "Attributes"
  Commodity_49 : Subsystem  mask{Mean=2000/84, AttributeValue=[6  12   4   0   0   0]|6|4|1}
      mask prompts: Mean "Frequency"; AttributeValue "Attributes"
  Commodity_50 : Subsystem  mask{Mean=2000/495, AttributeValue=[6  12   5   0   0   0]|6|5|1}
      mask prompts: Mean "Frequency"; AttributeValue "Attributes"
  Commodity_51 : Subsystem  mask{Mean=2000/443, AttributeValue=[6  12   7   0   0   0]|6|7|1}
      mask prompts: Mean "Frequency"; AttributeValue "Attributes"
  Commodity_52 : Subsystem  mask{Mean=2000/78, AttributeValue=[6  12  15   8   0   0]|6|8|1}
      mask prompts: Mean "Frequency"; AttributeValue "Attributes"
  Commodity_53 : Subsystem  mask{Mean=2000/204, AttributeValue=[6  12  15   9   0   0]|6|9|1}
      mask prompts: Mean "Frequency"; AttributeValue "Attributes"
  Commodity_54 : Subsystem  mask{Mean=2000/413, AttributeValue=[6  12  10   0   0   0]|6|10|1}
      mask prompts: Mean "Frequency"; AttributeValue "Attributes"
  Entity Sink : EntitySink
  Get Attribute : GetAttribute  AttributeName=Origin|Destination|Start  AttributeMissing=Error|Error|Error  AttributeDefaultValue=1|1|1  AttributeTreatAsVector=1|1|1  AttributeSendTiming=After entity departure|After entity departure|After entity departure  EvaluatedDefaultAttributeValue={[];[];[]}
      settings: OutputPortMap=o1,o2,o3
  Get Attribute1 : GetAttribute  AttributeName=Route  EvaluatedDefaultAttributeValue={[]}
      settings: OutputPortMap=o1
  IN_Commodity : PathCombiner  NumberInputPorts=9
  IN_Shipment : PathCombiner  NumberInputPorts=1
  Lookup : Constant  Value=[12]
  MATLAB Function : MATLAB Function  TreatAsAtomicUnit=on
  Mux : Mux  Inputs=3
  Node_ID : Constant  Value=6
  OUT_Shipment : OutputSwitch  NumberOutputPorts=1  SwitchingCriterion=From signal port p  AttributeName=Customer
  Shipment_Metrics : simeventslib/SimEvents Sinks/Discrete Event Signal to Workspace  VariableName=Customer_6  SaveFormat=Structure With Time  isMonitorOnly=off  isRecordIC=off
  Single Server : SingleServer  ServiceTime=0
  Timed to Evnt Signal : TimedToEventSignal
  Timed to Evnt Signal1 : TimedToEventSignal
  IN_Shipment_1 : PMIOPort  Port=1  Side=Left
  OUT_Shipment_1 : PMIOPort  Port=2  Side=Right
  wires:
  Timed to Evnt Signal1/1 -> MATLAB Function/3(lookup)
  Lookup/1 -> Timed to Evnt Signal1/1
  Timed to Evnt Signal/1 -> MATLAB Function/2(current)
  Get Attribute1/1 -> MATLAB Function/1(route)
  MATLAB Function/1(next) -> OUT_Shipment/1
  Node_ID/1 -> Timed to Evnt Signal/1
  Mux/1 -> Shipment_Metrics/1
  Get Attribute/3 -> Mux/3
  Get Attribute/2 -> Mux/2
  Get Attribute/1 -> Mux/1
  connections:
  Single Server/RConn1 -- OUT_Shipment/LConn1
  Get Attribute1/RConn1 -- Single Server/LConn1
  IN_Commodity/RConn1 -- Get Attribute1/LConn1
  Get Attribute/LConn1 -- IN_Shipment/RConn1
  Entity Sink/LConn1 -- Get Attribute/RConn1
  IN_Shipment/LConn1 -- IN_Shipment_1/RConn1
  OUT_Shipment/RConn1 -- OUT_Shipment_1/RConn1
  Commodity_46/RConn1 -- IN_Commodity/LConn1
  Commodity_47/RConn1 -- IN_Commodity/LConn2
  Commodity_48/RConn1 -- IN_Commodity/LConn3
  Commodity_49/RConn1 -- IN_Commodity/LConn4
  Commodity_50/RConn1 -- IN_Commodity/LConn5
  Commodity_51/RConn1 -- IN_Commodity/LConn6
  Commodity_52/RConn1 -- IN_Commodity/LConn7
  Commodity_53/RConn1 -- IN_Commodity/LConn8
  Commodity_54/RConn1 -- IN_Commodity/LConn9

== system Distribution_vAggregate/Customer_7 ==
  Commodity_55 : Subsystem  mask{Mean=2000/160, AttributeValue=[7  12  17   1   0   0]|7|1|1}
      mask prompts: Mean "Frequency"; AttributeValue "Attributes"
  Commodity_56 : Subsystem  mask{Mean=2000/45, AttributeValue=[7  12  15   2   0   0]|7|2|1}
      mask prompts: Mean "Frequency"; AttributeValue "Attributes"
  Commodity_57 : Subsystem  mask{Mean=2000/69, AttributeValue=[7  12  15   3   0   0]|7|3|1}
      mask prompts: Mean "Frequency"; AttributeValue "Attributes"
  Commodity_58 : Subsystem  mask{Mean=2000/248, AttributeValue=[7  12   4   0   0   0]|7|4|1}
      mask prompts: Mean "Frequency"; AttributeValue "Attributes"
  Commodity_59 : Subsystem  mask{Mean=2000/248, AttributeValue=[7  12   5   0   0   0]|7|5|1}
      mask prompts: Mean "Frequency"; AttributeValue "Attributes"
  Commodity_60 : Subsystem  mask{Mean=2000/28, AttributeValue=[7  12   6   0   0   0]|7|6|1}
      mask prompts: Mean "Frequency"; AttributeValue "Attributes"
  Commodity_61 : Subsystem  mask{Mean=2000/281, AttributeValue=[7  12  15   8   0   0]|7|8|1}
      mask prompts: Mean "Frequency"; AttributeValue "Attributes"
  Commodity_62 : Subsystem  mask{Mean=2000/349, AttributeValue=[7  12  15   9   0   0]|7|9|1}
      mask prompts: Mean "Frequency"; AttributeValue "Attributes"
  Commodity_63 : Subsystem  mask{Mean=2000/408, AttributeValue=[7  12  10   0   0   0]|7|10|1}
      mask prompts: Mean "Frequency"; AttributeValue "Attributes"
  Entity Sink : EntitySink
  Get Attribute : GetAttribute  AttributeName=Origin|Destination|Start  AttributeMissing=Error|Error|Error  AttributeDefaultValue=1|1|1  AttributeTreatAsVector=1|1|1  AttributeSendTiming=After entity departure|After entity departure|After entity departure  EvaluatedDefaultAttributeValue={[];[];[]}
      settings: OutputPortMap=o1,o2,o3
  Get Attribute1 : GetAttribute  AttributeName=Route  EvaluatedDefaultAttributeValue={[]}
      settings: OutputPortMap=o1
  IN_Commodity : PathCombiner  NumberInputPorts=9
  IN_Shipment : PathCombiner  NumberInputPorts=1
  Lookup : Constant  Value=[12]
  MATLAB Function : MATLAB Function  TreatAsAtomicUnit=on
  Mux : Mux  Inputs=3
  Node_ID : Constant  Value=7
  OUT_Shipment : OutputSwitch  NumberOutputPorts=1  SwitchingCriterion=From signal port p  AttributeName=Customer
  Shipment_Metrics : simeventslib/SimEvents Sinks/Discrete Event Signal to Workspace  VariableName=Customer_7  SaveFormat=Structure With Time  isMonitorOnly=off  isRecordIC=off
  Single Server : SingleServer  ServiceTime=0
  Timed to Evnt Signal : TimedToEventSignal
  Timed to Evnt Signal1 : TimedToEventSignal
  IN_Shipment_1 : PMIOPort  Port=1  Side=Left
  OUT_Shipment_1 : PMIOPort  Port=2  Side=Right
  wires:
  Timed to Evnt Signal1/1 -> MATLAB Function/3(lookup)
  Lookup/1 -> Timed to Evnt Signal1/1
  Timed to Evnt Signal/1 -> MATLAB Function/2(current)
  Get Attribute1/1 -> MATLAB Function/1(route)
  MATLAB Function/1(next) -> OUT_Shipment/1
  Node_ID/1 -> Timed to Evnt Signal/1
  Mux/1 -> Shipment_Metrics/1
  Get Attribute/3 -> Mux/3
  Get Attribute/2 -> Mux/2
  Get Attribute/1 -> Mux/1
  connections:
  Single Server/RConn1 -- OUT_Shipment/LConn1
  Get Attribute1/RConn1 -- Single Server/LConn1
  IN_Commodity/RConn1 -- Get Attribute1/LConn1
  Get Attribute/LConn1 -- IN_Shipment/RConn1
  Entity Sink/LConn1 -- Get Attribute/RConn1
  IN_Shipment/LConn1 -- IN_Shipment_1/RConn1
  OUT_Shipment/RConn1 -- OUT_Shipment_1/RConn1
  Commodity_55/RConn1 -- IN_Commodity/LConn1
  Commodity_56/RConn1 -- IN_Commodity/LConn2
  Commodity_57/RConn1 -- IN_Commodity/LConn3
  Commodity_58/RConn1 -- IN_Commodity/LConn4
  Commodity_59/RConn1 -- IN_Commodity/LConn5
  Commodity_60/RConn1 -- IN_Commodity/LConn6
  Commodity_61/RConn1 -- IN_Commodity/LConn7
  Commodity_62/RConn1 -- IN_Commodity/LConn8
  Commodity_63/RConn1 -- IN_Commodity/LConn9

== system Distribution_vAggregate/Customer_8 ==
  Commodity_64 : Subsystem  mask{Mean=2000/495, AttributeValue=[8  15  17   1   0   0]|8|1|1}
      mask prompts: Mean "Frequency"; AttributeValue "Attributes"
  Commodity_65 : Subsystem  mask{Mean=2000/433, AttributeValue=[8  15   2   0   0   0]|8|2|1}
      mask prompts: Mean "Frequency"; AttributeValue "Attributes"
  Commodity_66 : Subsystem  mask{Mean=2000/495, AttributeValue=[8  15   3   0   0   0]|8|3|1}
      mask prompts: Mean "Frequency"; AttributeValue "Attributes"
  Commodity_67 : Subsystem  mask{Mean=2000/240, AttributeValue=[8  15  12   4   0   0]|8|4|1}
      mask prompts: Mean "Frequency"; AttributeValue "Attributes"
  Commodity_68 : Subsystem  mask{Mean=2000/114, AttributeValue=[8  15  12   5   0   0]|8|5|1}
      mask prompts: Mean "Frequency"; AttributeValue "Attributes"
  Commodity_69 : Subsystem  mask{Mean=2000/451, AttributeValue=[8  15  12   6   0   0]|8|6|1}
      mask prompts: Mean "Frequency"; AttributeValue "Attributes"
  Commodity_70 : Subsystem  mask{Mean=2000/423, AttributeValue=[8  15  12   7   0   0]|8|7|1}
      mask prompts: Mean "Frequency"; AttributeValue "Attributes"
  Commodity_71 : Subsystem  mask{Mean=2000/293, AttributeValue=[8  15   9   0   0   0]|8|9|1}
      mask prompts: Mean "Frequency"; AttributeValue "Attributes"
  Commodity_72 : Subsystem  mask{Mean=2000/334, AttributeValue=[8  15  12  10   0   0]|8|10|1}
      mask prompts: Mean "Frequency"; AttributeValue "Attributes"
  Entity Sink : EntitySink
  Get Attribute : GetAttribute  AttributeName=Origin|Destination|Start  AttributeMissing=Error|Error|Error  AttributeDefaultValue=1|1|1  AttributeTreatAsVector=1|1|1  AttributeSendTiming=After entity departure|After entity departure|After entity departure  EvaluatedDefaultAttributeValue={[];[];[]}
      settings: OutputPortMap=o1,o2,o3
  Get Attribute1 : GetAttribute  AttributeName=Route  EvaluatedDefaultAttributeValue={[]}
      settings: OutputPortMap=o1
  IN_Commodity : PathCombiner  NumberInputPorts=9
  IN_Shipment : PathCombiner  NumberInputPorts=1
  Lookup : Constant  Value=[15]
  MATLAB Function : MATLAB Function  TreatAsAtomicUnit=on
  Mux : Mux  Inputs=3
  Node_ID : Constant  Value=8
  OUT_Shipment : OutputSwitch  NumberOutputPorts=1  SwitchingCriterion=From signal port p  AttributeName=Customer
  Shipment_Metrics : simeventslib/SimEvents Sinks/Discrete Event Signal to Workspace  VariableName=Customer_8  SaveFormat=Structure With Time  isMonitorOnly=off  isRecordIC=off
  Single Server : SingleServer  ServiceTime=0
  Timed to Evnt Signal : TimedToEventSignal
  Timed to Evnt Signal1 : TimedToEventSignal
  IN_Shipment_1 : PMIOPort  Port=1  Side=Left
  OUT_Shipment_1 : PMIOPort  Port=2  Side=Right
  wires:
  Timed to Evnt Signal1/1 -> MATLAB Function/3(lookup)
  Lookup/1 -> Timed to Evnt Signal1/1
  Timed to Evnt Signal/1 -> MATLAB Function/2(current)
  Get Attribute1/1 -> MATLAB Function/1(route)
  MATLAB Function/1(next) -> OUT_Shipment/1
  Node_ID/1 -> Timed to Evnt Signal/1
  Mux/1 -> Shipment_Metrics/1
  Get Attribute/3 -> Mux/3
  Get Attribute/2 -> Mux/2
  Get Attribute/1 -> Mux/1
  connections:
  Single Server/RConn1 -- OUT_Shipment/LConn1
  Get Attribute1/RConn1 -- Single Server/LConn1
  IN_Commodity/RConn1 -- Get Attribute1/LConn1
  Get Attribute/LConn1 -- IN_Shipment/RConn1
  Entity Sink/LConn1 -- Get Attribute/RConn1
  IN_Shipment/LConn1 -- IN_Shipment_1/RConn1
  OUT_Shipment/RConn1 -- OUT_Shipment_1/RConn1
  Commodity_64/RConn1 -- IN_Commodity/LConn1
  Commodity_65/RConn1 -- IN_Commodity/LConn2
  Commodity_66/RConn1 -- IN_Commodity/LConn3
  Commodity_67/RConn1 -- IN_Commodity/LConn4
  Commodity_68/RConn1 -- IN_Commodity/LConn5
  Commodity_69/RConn1 -- IN_Commodity/LConn6
  Commodity_70/RConn1 -- IN_Commodity/LConn7
  Commodity_71/RConn1 -- IN_Commodity/LConn8
  Commodity_72/RConn1 -- IN_Commodity/LConn9

== system Distribution_vAggregate/Customer_9 ==
  Commodity_73 : Subsystem  mask{Mean=2000/313, AttributeValue=[9  15  17   1   0   0]|9|1|1}
      mask prompts: Mean "Frequency"; AttributeValue "Attributes"
  Commodity_74 : Subsystem  mask{Mean=2000/365, AttributeValue=[9  15   2   0   0   0]|9|2|1}
      mask prompts: Mean "Frequency"; AttributeValue "Attributes"
  Commodity_75 : Subsystem  mask{Mean=2000/492, AttributeValue=[9  15   3   0   0   0]|9|3|1}
      mask prompts: Mean "Frequency"; AttributeValue "Attributes"
  Commodity_76 : Subsystem  mask{Mean=2000/291, AttributeValue=[9  15  12   4   0   0]|9|4|1}
      mask prompts: Mean "Frequency"; AttributeValue "Attributes"
  Commodity_77 : Subsystem  mask{Mean=2000/291, AttributeValue=[9  15  12   5   0   0]|9|5|1}
      mask prompts: Mean "Frequency"; AttributeValue "Attributes"
  Commodity_78 : Subsystem  mask{Mean=2000/61, AttributeValue=[9  15  12   6   0   0]|9|6|1}
      mask prompts: Mean "Frequency"; AttributeValue "Attributes"
  Commodity_79 : Subsystem  mask{Mean=2000/243, AttributeValue=[9  15  12   7   0   0]|9|7|1}
      mask prompts: Mean "Frequency"; AttributeValue "Attributes"
  Commodity_80 : Subsystem  mask{Mean=2000/105, AttributeValue=[9  15   8   0   0   0]|9|8|1}
      mask prompts: Mean "Frequency"; AttributeValue "Attributes"
  Commodity_81 : Subsystem  mask{Mean=2000/315, AttributeValue=[9  15  12  10   0   0]|9|10|1}
      mask prompts: Mean "Frequency"; AttributeValue "Attributes"
  Entity Sink : EntitySink
  Get Attribute : GetAttribute  AttributeName=Origin|Destination|Start  AttributeMissing=Error|Error|Error  AttributeDefaultValue=1|1|1  AttributeTreatAsVector=1|1|1  AttributeSendTiming=After entity departure|After entity departure|After entity departure  EvaluatedDefaultAttributeValue={[];[];[]}
      settings: OutputPortMap=o1,o2,o3
  Get Attribute1 : GetAttribute  AttributeName=Route  EvaluatedDefaultAttributeValue={[]}
      settings: OutputPortMap=o1
  IN_Commodity : PathCombiner  NumberInputPorts=9
  IN_Shipment : PathCombiner  NumberInputPorts=1
  Lookup : Constant  Value=[15]
  MATLAB Function : MATLAB Function  TreatAsAtomicUnit=on
  Mux : Mux  Inputs=3
  Node_ID : Constant  Value=9
  OUT_Shipment : OutputSwitch  NumberOutputPorts=1  SwitchingCriterion=From signal port p  AttributeName=Customer
  Shipment_Metrics : simeventslib/SimEvents Sinks/Discrete Event Signal to Workspace  VariableName=Customer_9  SaveFormat=Structure With Time  isMonitorOnly=off  isRecordIC=off
  Single Server : SingleServer  ServiceTime=0
  Timed to Evnt Signal : TimedToEventSignal
  Timed to Evnt Signal1 : TimedToEventSignal
  IN_Shipment_1 : PMIOPort  Port=1  Side=Left
  OUT_Shipment_1 : PMIOPort  Port=2  Side=Right
  wires:
  Timed to Evnt Signal1/1 -> MATLAB Function/3(lookup)
  Lookup/1 -> Timed to Evnt Signal1/1
  Timed to Evnt Signal/1 -> MATLAB Function/2(current)
  Get Attribute1/1 -> MATLAB Function/1(route)
  MATLAB Function/1(next) -> OUT_Shipment/1
  Node_ID/1 -> Timed to Evnt Signal/1
  Mux/1 -> Shipment_Metrics/1
  Get Attribute/3 -> Mux/3
  Get Attribute/2 -> Mux/2
  Get Attribute/1 -> Mux/1
  connections:
  Single Server/RConn1 -- OUT_Shipment/LConn1
  Get Attribute1/RConn1 -- Single Server/LConn1
  IN_Commodity/RConn1 -- Get Attribute1/LConn1
  Get Attribute/LConn1 -- IN_Shipment/RConn1
  Entity Sink/LConn1 -- Get Attribute/RConn1
  IN_Shipment/LConn1 -- IN_Shipment_1/RConn1
  OUT_Shipment/RConn1 -- OUT_Shipment_1/RConn1
  Commodity_73/RConn1 -- IN_Commodity/LConn1
  Commodity_74/RConn1 -- IN_Commodity/LConn2
  Commodity_75/RConn1 -- IN_Commodity/LConn3
  Commodity_76/RConn1 -- IN_Commodity/LConn4
  Commodity_77/RConn1 -- IN_Commodity/LConn5
  Commodity_78/RConn1 -- IN_Commodity/LConn6
  Commodity_79/RConn1 -- IN_Commodity/LConn7
  Commodity_80/RConn1 -- IN_Commodity/LConn8
  Commodity_81/RConn1 -- IN_Commodity/LConn9

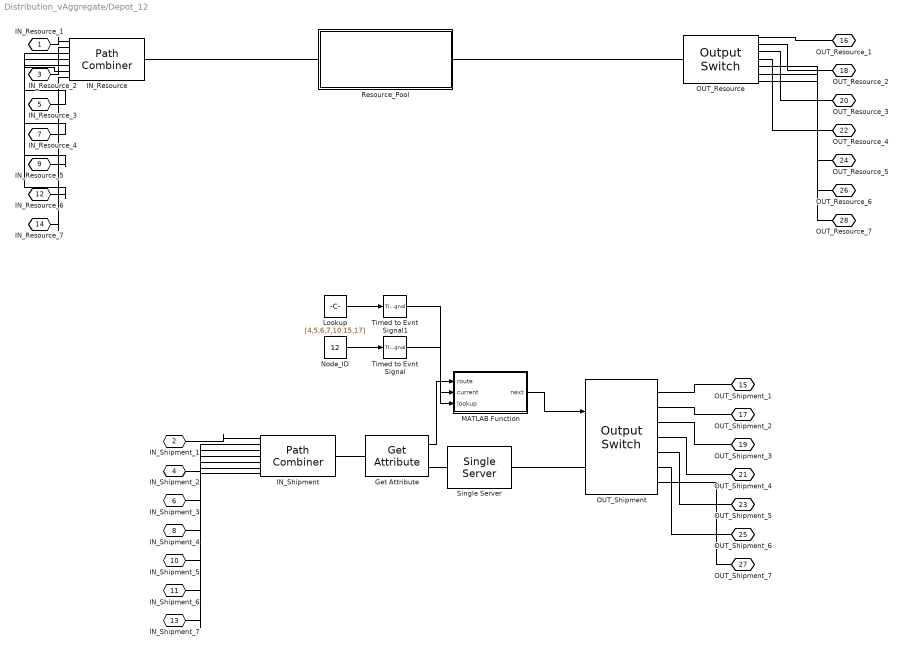
== system Distribution_vAggregate/Depot_12 ==
  Get Attribute : GetAttribute  AttributeName=Route  EvaluatedDefaultAttributeValue={[]}
      settings: OutputPortMap=o1
  IN_Resource : PathCombiner  NumberInputPorts=7
  IN_Shipment : PathCombiner  NumberInputPorts=7
  Lookup : Constant  Value=[4,5,6,7,10,15,17]
  MATLAB Function : MATLAB Function  TreatAsAtomicUnit=on
  Node_ID : Constant  Value=12
  OUT_Resource : OutputSwitch  NumberOutputPorts=7  SwitchingCriterion=Round robin  InitialSeed=57769
  OUT_Shipment : OutputSwitch  NumberOutputPorts=7  SwitchingCriterion=From signal port p  AttributeName=Customer
  Resource_Pool : Subsystem  mask{Quantity=6}
      mask prompts: Quantity "How many entities in resource pool?"
  Single Server : SingleServer  ServiceTime=0
  Timed to Evnt Signal : TimedToEventSignal
  Timed to Evnt Signal1 : TimedToEventSignal
  IN_Resource_1 : PMIOPort  Port=1  Side=Left
  IN_Shipment_1 : PMIOPort  Port=2  Side=Left
  IN_Resource_2 : PMIOPort  Port=3  Side=Left
  IN_Shipment_2 : PMIOPort  Port=4  Side=Left
  IN_Resource_3 : PMIOPort  Port=5  Side=Left
  IN_Shipment_3 : PMIOPort  Port=6  Side=Left
  IN_Resource_4 : PMIOPort  Port=7  Side=Left
  IN_Shipment_4 : PMIOPort  Port=8  Side=Left
  IN_Resource_5 : PMIOPort  Port=9  Side=Left
  IN_Shipment_5 : PMIOPort  Port=10  Side=Left
  IN_Shipment_6 : PMIOPort  Port=11  Side=Left
  IN_Resource_6 : PMIOPort  Port=12  Side=Left
  IN_Shipment_7 : PMIOPort  Port=13  Side=Left
  IN_Resource_7 : PMIOPort  Port=14  Side=Left
  OUT_Shipment_1 : PMIOPort  Port=15  Side=Right
  OUT_Resource_1 : PMIOPort  Port=16  Side=Right
  OUT_Shipment_2 : PMIOPort  Port=17  Side=Right
  OUT_Resource_2 : PMIOPort  Port=18  Side=Right
  OUT_Shipment_3 : PMIOPort  Port=19  Side=Right
  OUT_Resource_3 : PMIOPort  Port=20  Side=Right
  OUT_Shipment_4 : PMIOPort  Port=21  Side=Right
  OUT_Resource_4 : PMIOPort  Port=22  Side=Right
  OUT_Shipment_5 : PMIOPort  Port=23  Side=Right
  OUT_Resource_5 : PMIOPort  Port=24  Side=Right
  OUT_Shipment_6 : PMIOPort  Port=25  Side=Right
  OUT_Resource_6 : PMIOPort  Port=26  Side=Right
  OUT_Shipment_7 : PMIOPort  Port=27  Side=Right
  OUT_Resource_7 : PMIOPort  Port=28  Side=Right
  wires:
  Timed to Evnt Signal1/1 -> MATLAB Function/3(lookup)
  Lookup/1 -> Timed to Evnt Signal1/1
  Timed to Evnt Signal/1 -> MATLAB Function/2(current)
  Get Attribute/1 -> MATLAB Function/1(route)
  MATLAB Function/1(next) -> OUT_Shipment/1
  Node_ID/1 -> Timed to Evnt Signal/1
  connections:
  Resource_Pool/LConn1 -- OUT_Resource/LConn1
  Single Server/RConn1 -- OUT_Shipment/LConn1
  Get Attribute/RConn1 -- Single Server/LConn1
  IN_Shipment/RConn1 -- Get Attribute/LConn1
  Resource_Pool/RConn1 -- IN_Resource/RConn1
  IN_Resource/LConn1 -- IN_Resource_1/RConn1
  IN_Resource/LConn2 -- IN_Resource_2/RConn1
  IN_Resource/LConn3 -- IN_Resource_3/RConn1
  IN_Resource/LConn4 -- IN_Resource_4/RConn1
  IN_Resource/LConn5 -- IN_Resource_5/RConn1
  IN_Resource/LConn6 -- IN_Resource_6/RConn1
  IN_Resource/LConn7 -- IN_Resource_7/RConn1
  OUT_Resource/RConn1 -- OUT_Resource_1/RConn1
  OUT_Resource/RConn2 -- OUT_Resource_2/RConn1
  OUT_Resource/RConn3 -- OUT_Resource_3/RConn1
  OUT_Resource/RConn4 -- OUT_Resource_4/RConn1
  OUT_Resource/RConn5 -- OUT_Resource_5/RConn1
  OUT_Resource/RConn6 -- OUT_Resource_6/RConn1
  OUT_Resource/RConn7 -- OUT_Resource_7/RConn1
  IN_Shipment/LConn1 -- IN_Shipment_1/RConn1
  IN_Shipment/LConn2 -- IN_Shipment_2/RConn1
  IN_Shipment/LConn3 -- IN_Shipment_3/RConn1
  IN_Shipment/LConn4 -- IN_Shipment_4/RConn1
  IN_Shipment/LConn5 -- IN_Shipment_5/RConn1
  IN_Shipment/LConn6 -- IN_Shipment_6/RConn1
  IN_Shipment/LConn7 -- IN_Shipment_7/RConn1
  OUT_Shipment/RConn1 -- OUT_Shipment_1/RConn1
  OUT_Shipment/RConn2 -- OUT_Shipment_2/RConn1
  OUT_Shipment/RConn3 -- OUT_Shipment_3/RConn1
  OUT_Shipment/RConn4 -- OUT_Shipment_4/RConn1
  OUT_Shipment/RConn5 -- OUT_Shipment_5/RConn1
  OUT_Shipment/RConn6 -- OUT_Shipment_6/RConn1
  OUT_Shipment/RConn7 -- OUT_Shipment_7/RConn1
